simulink model "LQG"  (R2019b)
settings: Solver=FixedStepAuto  StartTime=0.0  StopTime=50  FixedStep=.0001  RelTol=1e-3
values from neighbouring files (symbols this model uses):
  Fes = F-L*H    [KF3_Script.m]    (also in KF_Script.m; LQG_Script.m)
  K = dlqr(F(1:2,1:2),G(1:2),[1 0;0 .1],0.01)    [LQG_Script.m]
  Kt = 0.071    [KF3_Script.m]    (also in KF_Script.m; LQG_Script.m)
  L = (dlqr(F',H',Q,R))'    [KF3_Script.m]    (also in KF_Script.m; LQG_Script.m)
undefined symbols (not defined in the file or in its folder): G
libraries: simulink x2
settings Model: Creator=oboe  LastModifiedBy=Luca
settings DataIOCC: LimitDataPoints=on  SaveFormat=Array  ReturnWorkspaceOutputs=off
settings OptimizationCC: LifeSpan=inf
settings DebuggingCC: SolverPrmCheckMsg=warning  SFUnexpectedBacktrackingDiag=warning  SFNoUnconditionalDefaultTransitionDiag=warning  SFExecutionAtInitializationDiag=none  ArithmeticOperatorsInVariantConditions=warning
settings HardwareCC: ProdBitPerPointer=32  ProdBitPerSizeT=32  ProdBitPerPtrDiffT=32  ProdLargestAtomicFloat=None  ProdIntDivRoundTo=Undefined  ProdEndianess=Unspecified  ProdWordSize=32  ProdHWDeviceType=32-bit Generic
settings ModelReferenceCC: PropagateSignalLabelsOutOfModel=off
settings SFSimCC: SimUseLocalCustomCode=off  CustomCodeUndefinedFunction=UseInterfaceOnly
settings RTWCC: RTWUseLocalCustomCode=off
settings CodeAppCC: StateflowObjectComments=on
settings GRTTargetCC: TargetLangStandard=C89/C90 (ANSI)
settings ConfigComp: CovMetricSettings=dw  CovHtmlReporting=on  CovSaveCumulativeToWorkspaceVar=on  CovSaveSingleToWorkspaceVar=on  CovExternalEMLEnable=off  CovSFcnEnable=off

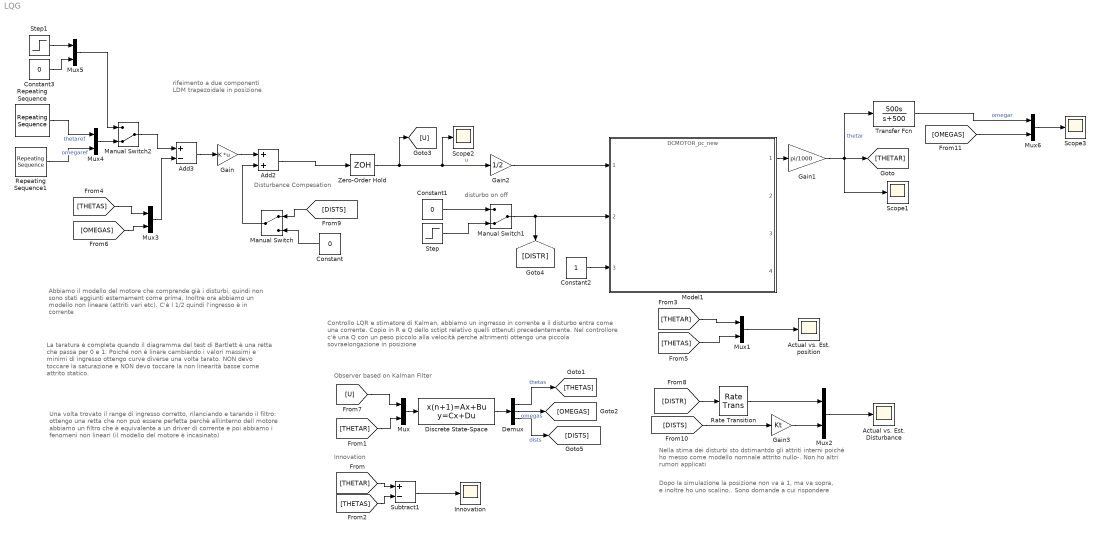
== system LQG ==
  note: Observer based on Kalman Filter
  note: Innovation
  note: Disturbance Compesation
  note: Controllo LQR e stimatore di Kalman, abbiamo un ingrresso in corrente e
      | il disturbo entra come una corrente. Copio in R e Q dello sctipt relativo quelli
      | ottenuti precedentemente.
      | Nel controllore c'è una Q con un peso piccolo alla velocità perche altrimenti
      | ottengo una piccola sovraelongazione in posizione
  note: Dopo la simulazione la posizione
      | non va a 1, ma va sopra, e inoltre ho
      | uno scalino.. Sono domande a cui rispondere
  note: Nella stima dei disturbi sto  dstimantdo gli attriti
      | interni poiché ho messo come modello nomnale
      | attrito nullo-. Non ho altri rumori applicati
  note: disturbo on off
  note: rifeimento a due componenti LDM trapezoidale in posizione
  note: Abbiamo il modello del motore che comprende già i disturbi, quindi non sono stati aggiunti esternament come prima, Inoltre ora
      | abbiamo un modello non lineare (attriti vari etc). C'è l 1/2 quindi l'ingresso è in corrente
  note: Una volta trovato il range di ingresso corretto, rilanciando
      | e tarando il filtro: ottengo una retta che non può essere
      | perfetta perchè allìinterno dell motore abbiamo un filtro che
      | è equivalente a un driver di corrente e poi abbiamo i fenomeni
      | non lineari (il modello del motore è incasinato)
  note: La taratura è completa quando il diagramma del test di
      | Bartlett è una retta che passa per 0 e 1. Poiché non è
      | linare cambiando i valori massimi e minimi di ingresso
      | ottengo curve diverse una volta tarato. NON devo toccare
      | la saturazione e NON devo toccare la non linearità basse
      | come attrito statico.
  Actual vs. Est. Disturbance : Scope
  Actual vs. Est. position : Scope
  Add2 : Sum
  Add3 : Sum  Inputs=+-
  Constant : Constant  Value=0
  Constant1 : Constant  Value=0
  Constant2 : Constant
  Constant3 : Constant  Value=0
  Demux : Demux  Outputs=3
  Discrete State-Space : DiscreteStateSpace  A=Fes  B=[G L]  C=eye(3)  D=zeros(3,2)  SampleTime=.001
  Gain : Gain  Gain=K  Multiplication=Matrix(K*u)
  Gain1 : Gain  Gain=pi/1000
  Gain2 : Gain  Gain=1/2
  Gain3 : Gain  Gain=Kt
  Innovation : Scope
  Manual Switch : ManualSwitch
  Manual Switch1 : ManualSwitch  CurrentSetting=0
  Manual Switch2 : ManualSwitch  CurrentSetting=0
  Model1 : ModelReference  ModelNameDialog=DCMOTOR_pc_new.slxp  ModelReferenceVersion=1.21  CopyOfModelProtected=on
  Mux{,1..6} (7 alike) : Mux  Inputs=2
  Rate Transition : RateTransition
  Repeating Sequence : simulink/Sources/Repeating Sequence  rep_seq_t=[0 1 2 3 4]  rep_seq_y=[0 0 1 1 0]*318*pi/1000
  Repeating Sequence1 : simulink/Sources/Repeating Sequence  rep_seq_t=[0 1-0.001 1 2-0.001 2 3-0.001 3 4-0.001 4]  rep_seq_y=[0 0 1 1 0 0 -1 -1 0]*318*pi/1000
  Scope1 : Scope
  Scope2 : Scope
  Scope3 : Scope
  Step : Step  After=.1  SampleTime=0
  Step1 : Step  Time=318*pi/2000  SampleTime=0
  Subtract1 : Sum  Inputs=+-
  Transfer Fcn : TransferFcn  Numerator=[500 0]  Denominator=[1 500]
  Zero-Order Hold : ZeroOrderHold  SampleTime=0.001
  wires:
  Mux/1 -> Discrete State-Space/1
  Discrete State-Space/1 -> Demux/1
  Demux/1 -> [THETAS]  "thetas"
  Mux1/1 -> Actual vs. Est. position/1
  Subtract1/1 -> Innovation/1
  Gain1/1 -> Transfer Fcn/1, Scope1/1, [THETAR]  "thetar"
  Gain/1 -> Add2/1
  Add2/1 -> Zero-Order Hold/1
  Demux/3 -> [DISTS]  "dists"
  Mux2/1 -> Actual vs. Est. Disturbance/1
  Demux/2 -> [OMEGAS]  "omegas"
  Repeating Sequence/1 -> Mux4/1  "thetaref"
  Repeating Sequence1/1 -> Mux4/2  "omegaref"
  Mux4/1 -> Manual Switch2/2
  Mux3/1 -> Add3/2
  Add3/1 -> Gain/1
  Manual Switch/1 -> Add2/2
  Constant/1 -> Manual Switch/2
  Constant1/1 -> Manual Switch1/1
  Step/1 -> Manual Switch1/2
  Model1/1 -> Gain1/1
  Zero-Order Hold/1 -> [U], Scope2/1, Gain2/1  "u"
  Gain2/1 -> Model1/1
  Manual Switch1/1 -> Model1/2, [DISTR]
  Gain3/1 -> Mux2/2
  Constant2/1 -> Model1/3
  Rate Transition/1 -> Mux2/1
  [THETAR] -> Subtract1/1
  [THETAR] -> Mux1/1
  [THETAR] -> Mux/2
  [THETAS] -> Subtract1/2
  [THETAS] -> Mux3/1
  [THETAS] -> Mux1/2
  [OMEGAS] -> Mux3/2
  [U] -> Mux/1
  [DISTR] -> Rate Transition/1
  [DISTS] -> Manual Switch/1
  [DISTS] -> Gain3/1
  Step1/1 -> Mux5/1
  Constant3/1 -> Mux5/2
  Manual Switch2/1 -> Add3/1
  Mux5/1 -> Manual Switch2/1
  Transfer Fcn/1 -> Mux6/1  "omegar"
  [OMEGAS] -> Mux6/2
  Mux6/1 -> Scope3/1
